simulink subsystem "mode_xOO"  (R2022a)
settings: Solver=VariableStepAuto  StartTime=0.0  StopTime=10.0  RelTol=1e-3
settings Model: Creator=bkfre  LastModifiedBy=bkfre

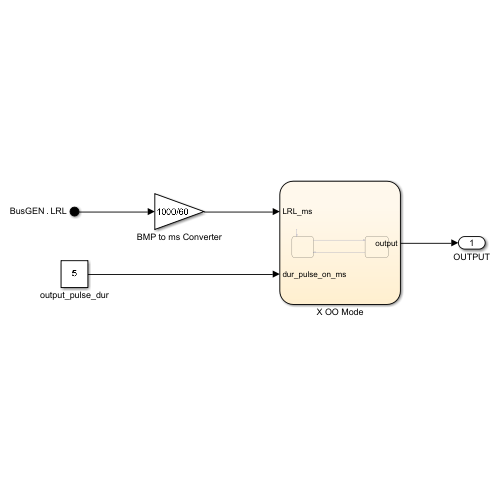
[thumbnail: Simulink's stored preview of the top-level diagram]
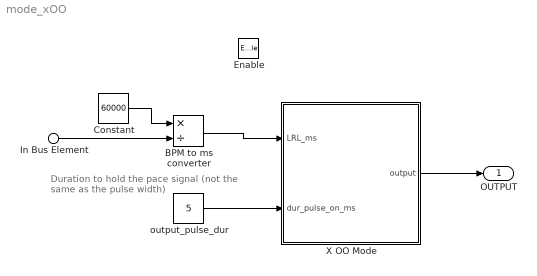
== system mode_xOO ==
  note: Duration to hold the pace signal (not the same as the pulse width)
  In Bus Element : Inport  PortName=BusGEN  Element=LRL
  Enable : EnablePort
  BPM to ms converter : Product  Inputs=*/
  Constant : Constant  Value=60000
  X OO Mode : Stateflow chart  TreatAsAtomicUnit=on
  output_pulse_dur : Constant  Value=5
  OUTPUT : Outport
  wires:
  X OO Mode/1(output) -> OUTPUT/1
  output_pulse_dur/1 -> X OO Mode/2(dur_pulse_on_ms)
  In Bus Element/1 -> BPM to ms converter/2
  BPM to ms converter/1 -> X OO Mode/1(LRL_ms)
  Constant/1 -> BPM to ms converter/1

== stateflow chart mode_xOO/X OO Mode ==
  note: Send a pace signal every LRL interval
  state Charge
    entry:
    output=0;
  state Pace
    entry:
    output=1;
  (default) -> Charge
  Charge -> Pace : after(LRL_ms-dur_pulse_on_ms,msec)
  Pace -> Charge : after(dur_pulse_on_ms,msec)
  data: LRL_ms input; dur_pulse_on_ms input; output output
